simulink model "VFlexP"  (R2024a)
settings: Solver=ode23tb  StartTime=0.0  StopTime=3  FixedStep=1e-5
model workspace (MAT data in the model file):
  DCop_DCBUCK : object (value not decoded)
  Grid_CCVSC_idx = [2; 3; 4; 5; 6; 7; 8; 9; 10; 11; 12]
  Grid_CCVSCs = 1
  Grid_CCVSCs_buses = 1
  Grid_CCVSCs_toM = [0 1 0 0 0 0 0 0 0 0 0 0 ... (781 elements, 71x11)]
  Grid_C_Lines = [0 0]
  Grid_Cbuses = [0.00666666666667 0.00666666666667 0.00666666666667]
  Grid_DC : object (value not decoded)
  Grid_DCop_DCBUCK : object (value not decoded)
  Grid_DCop_DC_PES : object (value not decoded)
  Grid_DFIGs = 1
  Grid_DFIGs_buses = 1
  Grid_DGs : string (value not decoded)
  Grid_From_buses = [1 2]
  Grid_GFls = 1
  Grid_GFls_buses = 1
  Grid_GFr_idx = 1
  Grid_GFrs = 1
  Grid_GFrs_buses = 1
  Grid_GFrs_toM = [1; 0; 0]
  Grid_IG_idx = 2
  Grid_IGs = 1
  Grid_IGs_buses = 1
  Grid_IGs_toM = [0; 1]
  Grid_L_Lines = [0.05 0.05]
  Grid_L_Loads = 0
  Grid_Lines_fromM : object (value not decoded)
  Grid_Lines_toM : object (value not decoded)
  Grid_Load_buses = []
  Grid_Load_busesDC = []
  Grid_MSGs = 1
  Grid_MSGs_buses = 1
  Grid_Nbuses = 3
  Grid_PQ_gen = 3
  Grid_Ploads = []
  Grid_PloadsDC = []
  Grid_Ps_lf = -0.138475313333
  Grid_Qloads = []
  Grid_Qs_lf = 0.00594619333333
  Grid_R_Lines = [0.005 0.005]
  Grid_R_Loads = 0
  Grid_R_Loads_DC = 0
  Grid_Rcf = [150 150 150]
  Grid_SCs = 1
  Grid_SCs_buses = 1
  Grid_SG_idx = 1
  Grid_SGs = 1
  Grid_SGs_buses = 1
  Grid_SGs_toM = [1; 0]
  Grid_To_buses = [2 3]
  Grid_VCVSC_idx = [1; 2; 3; 4; 5; 6; 7; 8; 9; 10; 11; 12]
  Grid_VCVSCs = 1
  Grid_VCVSCs_buses = [1; 2; 3; 6; 8; 9; 12; 58; 59; 60; 63; 65]
  Grid_VCVSCs_toM = [1 0 0 0 0 0 0 0 0 0 0 0 ... (852 elements, 71x12)]
  Grid_VSM_idx = 2
  Grid_VSMs = 1
  Grid_VSMs_buses = 1
  Grid_VSMs_toM = [0; 1]
  Grid_admitt_matrix = [1.9801990198-19.801979198i  -1.9801980198+19.801980198i; -1.9801980198+19.801980198i  1.9801990198-19.801979198i]
  Grid_admitt_matrix_noloads = [1.9801990198-19.801979198i  -1.9801980198+19.801980198i; -1.9801980198+19.801980198i  1.9801990198-19.801979198i]
  Grid_bus = [1; 2; 3]
  Grid_busDC_complexity = 1
  Grid_busDC_complexity_PF = 2
  Grid_bus_complexity = [1 1 1]
  Grid_bus_complexity_PF = [1 1 1]
  Grid_buses_lf = 1
  Grid_conductance_matrix = 0.00666666666667
  Grid_conductance_matrix_noloads = 0.00666666666667
  Grid_fref : object (value not decoded)
  Grid_gen_static_params : mBase (value not decoded)
  Grid_iPs_lf = -7.22150378958
  Grid_iQs_lf = 168.17482109
  Grid_iadmitt_matrix = [250000.001075-249999.987531i  249999.998575-250000.012531i; 249999.998575-250000.012531i  250000.001075-249999.987531i]
  Grid_iadmitt_matrix_noloads = [250000.001075-249999.987531i  249999.998575-250000.012531i; 249999.998575-250000.012531i  250000.001075-249999.987531i]
  Grid_iconductance_matrix = 150
  Grid_iconductance_matrix_noloads = 150
  Grid_init_OK_bool = 1
  Grid_intconv_PF : object (value not decoded)
  Grid_lf_op : op_report (value not decoded)
  Grid_lineDC_complexity = []
  Grid_lineDC_complexity_PF = []
  Grid_line_complexity = [1 1]
  Grid_line_complexity_PF = [3 3]
  Grid_loadDC_complexity = []
  Grid_loadDC_complexity_PF = []
  Grid_load_complexity = []
  Grid_load_complexity_PF = []
  Grid_opDC_CCVSC : object (value not decoded)
  Grid_opDC_VSM : object (value not decoded)
  Grid_opGFr : object (value not decoded)
  Grid_opVCVSC : object (value not decoded)
  Grid_op_CCVSC : object (value not decoded)
  Grid_op_IG : object (value not decoded)
  Grid_op_SG : object (value not decoded)
  Grid_op_VSM : object (value not decoded)
  Grid_shift_lines = [0 0]
  Grid_tap_lines = [1 1]
  Grid_v_buses_mod = [1 1.0001218564 1]
  LinsysParamChangeStruct : Param1 (value not decoded)
  Lline = 0.01
  Rline = 1e-05
  linsys : object (value not decoded)
symbols that are objects in the model workspace (value not decoded): Grid_DCop_DC_PES, Grid_DCop_DCBUCK, Grid_op_CCVSC, Grid_op_IG, Grid_op_SG, Grid_op_VSM, Grid_opDC_CCVSC, Grid_opDC_VSM, Grid_opGFr, Grid_opVCVSC
undefined symbols (not defined in the file or in its folder): block_buses_DC, block_idx, CCVSC_idx, Cf, costs, costs2, DFIGs_nodes, DiscIntNeverNeededParam, entity, Fb, Fi, From_nodes, Grid_op_DFIG, Grid_op_DFIG_PQ, Grid_op_MSG, Grid_op_SC, Grid_op_VCVSC, Kic, Kiv, Kpc, Kpv, last_send, Lc, Lf, m, Matrix_flux_to_i, mD, mp, MSGs_buses, Nbuses_DC, nq, op_VCVSC, Psche, Rc, Rf, rkq1, rkq2, SCs_buses, SCs_nodes, sec_control_structure, set_DG_up, set_extra_satur, set_sending_cost, SGs_buses, SGs_nodes, Tf, To_nodes, VI_L, VI_R, WOF_Tf, xkq1, xkq2
libraries: simulink x447, eeGeneralControl x5
(part 19 of 30)

== system VFlexP/Grid/Dynamic/Grid/Dynamic/Loads/PQ ==
  v_in : Inport
  connected : Inport  Port=2
  iP : Inport  Port=3
  Constant : Constant  Value=Ploads(load_complexity == 4)/Sb  VectorParams1D=off
  Constant1 : Constant  Value=Qloads(load_complexity == 4)/Sb  VectorParams1D=off
  Constant2 : Constant  Value=Inf
  Constant3 : Constant  Value=zeros(1, sum(load_complexity == 4))  VectorParams1D=off
  Divide : Product  Inputs=*/
  Divide1 : Product  Inputs=*/
  For Each Subsystem : Subsystem  TreatAsAtomicUnit=on
  Gain : Gain  Gain=Ploads(load_complexity == 4)/Sb
  Matrix Concatenate : Concatenate  NumInputs=3  Mode=Multidimensional array
  Product{,1..7} (8 alike) : Product
  Selector : Selector  NumberOfDimensions=2  InputPortWidth=3  IndexOptions=Index vector (dialog),Index vector (dialog)  Indices=1,find(load_complexity == 4)  OutputSizes=1,1
  Selector1 : Selector  NumberOfDimensions=2  InputPortWidth=3  IndexOptions=Index vector (dialog),Index vector (dialog)  Indices=2,find(load_complexity == 4)  OutputSizes=1,1
  Selector2 : Selector  InputPortWidth=length(R_Loads)  IndexOptions=Index vector (dialog)  Indices=find(load_complexity == 4)  OutputSizes=1
  Selector3 : Selector  InputPortWidth=length(R_Loads)  IndexOptions=Index vector (dialog)  Indices=find(load_complexity == 4)  OutputSizes=1
  Sum : Sum  Inputs=|++
  Sum1 : Sum  Inputs=|+-
  Sum2 : Sum  Inputs=|++
  Sum4 : Sum  Inputs=|++
  Switch : Switch  Criteria=u2 > Threshold  Threshold=1e-5  ZeroCross=off  SaturateOnIntegerOverflow=off  InputSameDT=off
  i : Outport
  wires:
  Product1/1 -> Sum/2
  Product/1 -> Sum/1
  Sum2/1 -> Product/1, Product2/1  "Prefnew"
  Product2/1 -> Sum1/1
  v_in/1 -> Selector1/1, Selector/1
  Product3/1 -> Sum1/2
  Product5/1 -> Sum4/2
  Constant1/1 -> Product3/1, Product1/2  "Qrefnew"
  Product4/1 -> Sum4/1
  Sum/1 -> Divide/1
  Switch/1 -> Divide1/2, Divide/2
  Sum4/1 -> Switch/1, Switch/2
  Constant2/1 -> Switch/3
  Sum1/1 -> Divide1/1
  connected/1 -> Selector2/1
  Divide/1 -> Product6/2  "id"
  Divide1/1 -> Product7/2  "iqref"
  Selector/1 -> Product4/1, Product4/2, Product/2, Product3/2  "id1"
  Selector1/1 -> Product5/1, Product5/2, Product2/2, Product1/1  "iq1"
  Matrix Concatenate/1 -> For Each Subsystem/1(In1)
  Product6/1 -> Matrix Concatenate/1
  Product7/1 -> Matrix Concatenate/2
  Selector2/1 -> Product6/1, Product7/1
  For Each Subsystem/1(Out1) -> i/1
  Constant3/1 -> Matrix Concatenate/3
  Selector3/1 -> Gain/1
  Gain/1 -> Sum2/1
  iP/1 -> Selector3/1
  Constant/1 -> Sum2/2  "Prefnew"

== system VFlexP/Grid/Dynamic/Grid/Dynamic/Loads/dynamic PQ ==
  v_in : Inport
  connected : Inport  Port=2
  iP : Inport  Port=3
  Constant : Constant  Value=Ploads(load_complexity == 5)/Sb  VectorParams1D=off
  Constant1 : Constant  Value=Qloads(load_complexity == 5)/Sb  VectorParams1D=off
  Constant2 : Constant  Value=Inf
  Constant3 : Constant  Value=zeros(1, sum(load_complexity == 5))  VectorParams1D=off
  Divide : Product  Inputs=*/
  Divide1 : Product  Inputs=*/
  For Each Subsystem : Subsystem  TreatAsAtomicUnit=on
  Gain : Gain  Gain=Ploads(load_complexity == 5)/Sb
  Matrix Concatenate : Concatenate  NumInputs=3  Mode=Multidimensional array
  Product{,1..7} (8 alike) : Product
  Selector : Selector  NumberOfDimensions=2  InputPortWidth=3  IndexOptions=Index vector (dialog),Index vector (dialog)  Indices=1,find(load_complexity == 5)  OutputSizes=1,1
  Selector1 : Selector  NumberOfDimensions=2  InputPortWidth=3  IndexOptions=Index vector (dialog),Index vector (dialog)  Indices=2,find(load_complexity == 5)  OutputSizes=1,1
  Selector2 : Selector  InputPortWidth=length(R_Loads)  IndexOptions=Index vector (dialog)  Indices=find(load_complexity == 5)  OutputSizes=1
  Selector3 : Selector  InputPortWidth=length(R_Loads)  IndexOptions=Index vector (dialog)  Indices=find(load_complexity == 5)  OutputSizes=1
  Signal Specification : SignalSpecification  Dimensions=[3 sum(load_complexity == 5)]
  Sum : Sum  Inputs=|++
  Sum1 : Sum  Inputs=|+-
  Sum2 : Sum  Inputs=|++
  Sum4 : Sum  Inputs=|++
  Switch : Switch  Criteria=u2 > Threshold  Threshold=1e-5  ZeroCross=off  SaturateOnIntegerOverflow=off  InputSameDT=off
  i_d : Subsystem  mask{T_s=0.01}
      mask prompts: T_s "Filter time constant"
      mask Display:
      | try
      |     dpoly(1, [T_s, 1])
      | catch
      | end
  i_q : Subsystem  mask{T_s=0.01}
      mask prompts: T_s "Filter time constant"
      mask Display:
      | try
      |     dpoly(1, [T_s, 1])
      | catch
      | end
  i : Outport
  wires:
  Product7/1 -> i_q/1(in)
  Divide1/1 -> Product7/2  "iqref"
  Product6/1 -> i_d/1(in)
  Divide/1 -> Product6/2  "id"
  connected/1 -> Selector2/1
  Sum1/1 -> Divide1/1
  Constant2/1 -> Switch/3
  Sum4/1 -> Switch/2, Switch/1
  Switch/1 -> Divide/2, Divide1/2
  Sum/1 -> Divide/1
  Product4/1 -> Sum4/1
  Product5/1 -> Sum4/2
  Product3/1 -> Sum1/2
  v_in/1 -> Selector/1, Selector1/1
  Product2/1 -> Sum1/1
  Sum2/1 -> Product2/1, Product/1  "Prefnew"
  Product/1 -> Sum/1
  Product1/1 -> Sum/2
  iP/1 -> Selector3/1
  Constant/1 -> Sum2/2  "Prefnew"
  Gain/1 -> Sum2/1
  Constant1/1 -> Product1/2, Product3/1  "Qrefnew"
  Selector/1 -> Product3/2, Product/2, Product4/2, Product4/1  "id1"
  Selector1/1 -> Product1/1, Product2/2, Product5/2, Product5/1  "iq1"
  Matrix Concatenate/1 -> Signal Specification/1
  i_d/1(out) -> Matrix Concatenate/1
  i_q/1(out) -> Matrix Concatenate/2
  Selector2/1 -> Product7/1, Product6/1
  Selector3/1 -> Gain/1
  For Each Subsystem/1(Out1) -> i/1
  Signal Specification/1 -> For Each Subsystem/1(In1)
  Constant3/1 -> Matrix Concatenate/3

== system VFlexP/Grid/Dynamic/Grid/Dynamic/Loads/parallel RL dynamic ==
  v_in : Inport
  connected : Inport  Port=2
  Constant : Constant
  Constant1 : Constant  Value=zeros(1, sum(load_complexity == 6))  VectorParams1D=off
  For Each Subsystem : Subsystem  TreatAsAtomicUnit=on
  Gain1 : Gain  Gain=(v_buses_mod(Load_buses(load_complexity == 6)).^2)./Qloads(load_complexity == 6)*Sb
  Gain2 : Gain  Gain=(Ploads(load_complexity == 6)./v_buses_mod(Load_buses(load_complexity == 6)).^2)/Sb
  Gain3 : Gain  Gain=(Ploads(load_complexity == 6)./v_buses_mod(Load_buses(load_complexity == 6)).^2)/Sb
  Gain4 : Gain  Gain=(v_buses_mod(Load_buses(load_complexity == 6)).^2)./Qloads(load_complexity == 6)*Sb
  Gain5 : Gain  Gain=Qloads(load_complexity == 6)./(v_buses_mod(Load_buses(load_complexity == 6)).^2)/Sb
  Gain7 : Gain  Gain=Qloads(load_complexity == 6)./(v_buses_mod(Load_buses(load_complexity == 6)).^2)/Sb
  Matrix Concatenate : Concatenate  NumInputs=3  Mode=Multidimensional array
  Product{,1,6..9} (6 alike) : Product
  Selector : Selector  NumberOfDimensions=2  InputPortWidth=3  IndexOptions=Index vector (dialog),Index vector (dialog)  Indices=1,find(load_complexity == 6)  OutputSizes=1,1
  Selector1 : Selector  NumberOfDimensions=2  InputPortWidth=3  IndexOptions=Index vector (dialog),Index vector (dialog)  Indices=2,find(load_complexity == 6)  OutputSizes=1,1
  Selector3 : Selector  InputPortWidth=length(R_Loads)  IndexOptions=Index vector (dialog)  Indices=find(load_complexity == 6)  OutputSizes=1
  Selector4 : Selector  InputPortWidth=length(fref.ref_units)  IndexOptions=Index vector (dialog)  Indices=fref.loads(load_complexity == 6)  OutputSizes=1
  Selector8 : Selector  InputPortWidth=length(fref.ref_units)  IndexOptions=Index vector (dialog)  Indices=fref.loads(load_complexity == 6)  OutputSizes=1
  Signal Specification : SignalSpecification  Dimensions=[3 sum(load_complexity == 6)]
  Sum : Sum  Inputs=|++
  Sum1 : Sum  Inputs=|++
  Sum6 : Sum  Inputs=|++
  Sum8 : Sum  Inputs=|+-
  i_d : Integrator  InitialCondition=Grid_lf_op.op_report.Outputs(8).y(Load_buses(load_complexity == 6)).*Qloads(load_complexity == 6)./(v_buses_mod(Load_buses(load_complexity == 6)).^2)/Sb
  i_q : Integrator  InitialCondition=Grid_lf_op.op_report.Outputs(7).y(Load_buses(load_complexity == 6)).*-Qloads(load_complexity == 6)./(v_buses_mod(Load_buses(load_complexity == 6)).^2)/Sb
  i : Outport
  wires:
  Sum8/1 -> Gain7/1
  Selector4/1 -> Product/2, Product1/1
  [omega_ref] -> Selector4/1  "omega"
  Signal Specification/1 -> For Each Subsystem/1(In1)
  Selector/1 -> Product8/2
  Product6/1 -> i_d/1
  Selector1/1 -> Product9/2
  Selector3/1 -> Product8/1, Product9/1
  i_q/1 -> Sum1/1, Gain4/1  "iq"
  connected/1 -> Selector3/1
  [omega_base] -> Selector8/1
  For Each Subsystem/1(Out1) -> i/1
  Gain1/1 -> Product1/2
  Sum6/1 -> Gain5/1
  Product1/1 -> Sum8/2
  Gain7/1 -> Product7/2
  i_d/1 -> Sum/1, Gain1/1  "id"
  Gain4/1 -> Product/1
  v_in/1 -> Selector/1, Selector1/1
  Product7/1 -> i_q/1
  Constant1/1 -> Matrix Concatenate/3
  Product/1 -> Sum6/2
  Selector8/1 -> Product7/1, Product6/2
  Product9/1 -> Gain3/1, Sum8/1
  Product8/1 -> Gain2/1, Sum6/1
  Matrix Concatenate/1 -> Signal Specification/1
  Gain5/1 -> Product6/1
  Sum/1 -> Matrix Concatenate/1
  Gain2/1 -> Sum/2
  Gain3/1 -> Sum1/2
  Sum1/1 -> Matrix Concatenate/2

== system VFlexP/Grid/Dynamic/Grid/Dynamic/Loads/parallel RL static ==
  v_in : Inport
  connected : Inport  Port=2
  Constant : Constant  Value=R_Loads(load_complexity == 1)  VectorParams1D=off
  Constant1 : Constant  Value=zeros(1, sum(load_complexity == 1))  VectorParams1D=off
  For Each Subsystem : Subsystem  TreatAsAtomicUnit=on
  Gain1 : Gain  Gain=L_Loads(load_complexity == 1)
  Gain4 : Gain  Gain=L_Loads(load_complexity == 1)
  Gain5 : Gain  Gain=1./L_Loads(load_complexity == 1)
  Gain7 : Gain  Gain=1./L_Loads(load_complexity == 1)
  Matrix Concatenate : Concatenate  NumInputs=3  Mode=Multidimensional array
  Product{,1,4..9} (8 alike) : Product
  Selector : Selector  NumberOfDimensions=2  InputPortWidth=3  IndexOptions=Index vector (dialog),Index vector (dialog)  Indices=1,find(load_complexity == 1)  OutputSizes=1,1
  Selector1 : Selector  NumberOfDimensions=2  InputPortWidth=3  IndexOptions=Index vector (dialog),Index vector (dialog)  Indices=2,find(load_complexity == 1)  OutputSizes=1,1
  Selector3 : Selector  InputPortWidth=length(R_Loads)  IndexOptions=Index vector (dialog)  Indices=find(load_complexity == 1)  OutputSizes=1
  Selector4 : Selector  InputPortWidth=length(fref.ref_units)  IndexOptions=Index vector (dialog)  Indices=fref.loads(load_complexity == 1)  OutputSizes=1
  Selector8 : Selector  InputPortWidth=length(fref.ref_units)  IndexOptions=Index vector (dialog)  Indices=fref.loads(load_complexity == 1)  OutputSizes=1
  Signal Specification : SignalSpecification  Dimensions=[3 sum(load_complexity == 1)]
  Sum4 : Sum  Inputs=+-|
  Sum5 : Sum  Inputs=|-+
  Sum6 : Sum  Inputs=|++
  Sum7 : Sum  Inputs=-+|
  Sum8 : Sum  Inputs=|+-
  Sum9 : Sum  Inputs=-+|
  Zero : Constant  Value=0  OutDataTypeStr=Inherit: Inherit via back propagation
  Zero1 : Constant  Value=0  OutDataTypeStr=Inherit: Inherit via back propagation
  i_d : Integrator  InitialCondition=Grid_lf_op.op_report.Outputs(5).y(load_complexity == 1)
  i_q : Integrator  InitialCondition=Grid_lf_op.op_report.Outputs(6).y(load_complexity == 1)
  i : Outport
  wires:
  v_in/1 -> Selector1/1, Selector/1
  Product5/1 -> Sum4/2
  i_d/1 -> Matrix Concatenate/1, Gain1/1, Product5/1  "id"
  Sum6/1 -> Gain5/1
  [omega_ref] -> Selector4/1  "omega"
  Product/1 -> Sum6/2
  Sum8/1 -> Gain7/1
  Sum4/1 -> Sum7/2
  Product1/1 -> Sum8/2
  Gain4/1 -> Product/1
  Sum7/1 -> Sum6/1
  Product4/1 -> Sum5/1
  Sum5/1 -> Sum9/2
  i_q/1 -> Matrix Concatenate/2, Product4/1, Gain4/1  "iq"
  Gain1/1 -> Product1/2
  Sum9/1 -> Sum8/1
  Zero/1 -> Sum7/1  "v_out_d"
  Zero1/1 -> Sum9/1  "v_out_q"
  Matrix Concatenate/1 -> Signal Specification/1
  Product8/1 -> Sum4/1  "id1"
  Product9/1 -> Sum5/2  "iq1"
  For Each Subsystem/1(Out1) -> i/1
  Signal Specification/1 -> For Each Subsystem/1(In1)
  Constant1/1 -> Matrix Concatenate/3
  Constant/1 -> Product5/2, Product4/2  "R"
  Selector4/1 -> Product1/1, Product/2
  [omega_base] -> Selector8/1
  Selector8/1 -> Product6/2, Product7/1
  Product7/1 -> i_q/1
  Gain7/1 -> Product7/2
  Gain5/1 -> Product6/1
  Product6/1 -> i_d/1
  connected/1 -> Selector3/1
  Selector/1 -> Product8/2  "id1"
  Selector3/1 -> Product9/1, Product8/1
  Selector1/1 -> Product9/2  "iq1"

== system VFlexP/Grid/Dynamic/Grid/Dynamic/Loads/parallel RL static omega ==
  v_in : Inport
  connected : Inport  Port=2
  Constant : Constant  Value=R_Loads(load_complexity == 1)  VectorParams1D=off
  Constant1 : Constant  Value=zeros(1, sum(load_complexity == 1))  VectorParams1D=off
  For Each Subsystem : Subsystem  TreatAsAtomicUnit=on
  Gain1 : Gain  Gain=L_Loads(load_complexity == 1)
  Gain4 : Gain  Gain=L_Loads(load_complexity == 1)
  Gain5 : Gain  Gain=1./L_Loads(load_complexity == 1)
  Gain7 : Gain  Gain=1./L_Loads(load_complexity == 1)
  Matrix Concatenate : Concatenate  NumInputs=3  Mode=Multidimensional array
  Product{,1,4..9} (8 alike) : Product
  Selector : Selector  NumberOfDimensions=2  InputPortWidth=3  IndexOptions=Index vector (dialog),Index vector (dialog)  Indices=1,find(load_complexity == 1)  OutputSizes=1,1
  Selector1 : Selector  NumberOfDimensions=2  InputPortWidth=3  IndexOptions=Index vector (dialog),Index vector (dialog)  Indices=2,find(load_complexity == 1)  OutputSizes=1,1
  Selector3 : Selector  InputPortWidth=length(R_Loads)  IndexOptions=Index vector (dialog)  Indices=find(load_complexity == 1)  OutputSizes=1
  Selector4 : Selector  InputPortWidth=length(fref.ref_units)  IndexOptions=Index vector (dialog)  Indices=fref.loads(load_complexity == 1)  OutputSizes=1
  Selector8 : Selector  InputPortWidth=length(fref.ref_units)  IndexOptions=Index vector (dialog)  Indices=fref.loads(load_complexity == 1)  OutputSizes=1
  Signal Specification : SignalSpecification  Dimensions=[3 sum(load_complexity == 1)]
  Sum4 : Sum  Inputs=+-|
  Sum5 : Sum  Inputs=|-+
  Sum6 : Sum  Inputs=|++
  Sum7 : Sum  Inputs=-+|
  Sum8 : Sum  Inputs=|+-
  Sum9 : Sum  Inputs=-+|
  Zero : Constant  Value=0  OutDataTypeStr=Inherit: Inherit via back propagation
  Zero1 : Constant  Value=0  OutDataTypeStr=Inherit: Inherit via back propagation
  i_d : Integrator  InitialCondition=Grid_lf_op.op_report.Outputs(5).y(load_complexity == 1)
  i_q : Integrator  InitialCondition=Grid_lf_op.op_report.Outputs(6).y(load_complexity == 1)
  i : Outport
  wires:
  Selector1/1 -> Product9/2  "iq1"
  Selector3/1 -> Product8/1, Product9/1
  Selector/1 -> Product8/2  "id1"
  connected/1 -> Selector3/1
  Product6/1 -> i_d/1
  Gain5/1 -> Product6/1
  Gain7/1 -> Product7/2
  Product7/1 -> i_q/1
  Selector8/1 -> Product7/1, Product6/2
  [omega_base] -> Selector8/1
  Selector4/1 -> Product/2, Product1/1
  Constant/1 -> Product4/2, Product5/2  "R"
  Constant1/1 -> Matrix Concatenate/3
  Signal Specification/1 -> For Each Subsystem/1(In1)
  For Each Subsystem/1(Out1) -> i/1
  Product9/1 -> Sum5/2  "iq1"
  Product8/1 -> Sum4/1  "id1"
  Matrix Concatenate/1 -> Signal Specification/1
  Zero1/1 -> Sum9/1  "v_out_q"
  Zero/1 -> Sum7/1  "v_out_d"
  Sum9/1 -> Sum8/1
  Gain1/1 -> Product1/2
  i_q/1 -> Gain4/1, Product4/1, Matrix Concatenate/2  "iq"
  Sum5/1 -> Sum9/2
  Product4/1 -> Sum5/1
  Sum7/1 -> Sum6/1
  Gain4/1 -> Product/1
  Product1/1 -> Sum8/2
  Sum4/1 -> Sum7/2
  Sum8/1 -> Gain7/1
  Product/1 -> Sum6/2
  [omega_ref] -> Selector4/1  "omega"
  Sum6/1 -> Gain5/1
  i_d/1 -> Product5/1, Gain1/1, Matrix Concatenate/1  "id"
  Product5/1 -> Sum4/2
  v_in/1 -> Selector/1, Selector1/1

== system VFlexP/Grid/Dynamic/Grid/Dynamic/Loads/series RL dynamic ==
  v_in : Inport
  connected : Inport  Port=2
  Constant : Constant  Value=R_Loads(load_complexity == 1)  VectorParams1D=off
  Constant1 : Constant  Value=zeros(1, sum(load_complexity == 1))  VectorParams1D=off
  For Each Subsystem : Subsystem  TreatAsAtomicUnit=on
  Gain1 : Gain  Gain=L_Loads(load_complexity == 1)
  Gain4 : Gain  Gain=L_Loads(load_complexity == 1)
  Gain5 : Gain  Gain=1./L_Loads(load_complexity == 1)
  Gain7 : Gain  Gain=1./L_Loads(load_complexity == 1)
  Matrix Concatenate : Concatenate  NumInputs=3  Mode=Multidimensional array
  Product{,1,4..9} (8 alike) : Product
  Selector : Selector  NumberOfDimensions=2  InputPortWidth=3  IndexOptions=Index vector (dialog),Index vector (dialog)  Indices=1,find(load_complexity == 1)  OutputSizes=1,1
  Selector1 : Selector  NumberOfDimensions=2  InputPortWidth=3  IndexOptions=Index vector (dialog),Index vector (dialog)  Indices=2,find(load_complexity == 1)  OutputSizes=1,1
  Selector3 : Selector  InputPortWidth=length(R_Loads)  IndexOptions=Index vector (dialog)  Indices=find(load_complexity == 1)  OutputSizes=1
  Selector4 : Selector  InputPortWidth=length(fref.ref_units)  IndexOptions=Index vector (dialog)  Indices=fref.loads(load_complexity == 1)  OutputSizes=1
  Selector8 : Selector  InputPortWidth=length(fref.ref_units)  IndexOptions=Index vector (dialog)  Indices=fref.loads(load_complexity == 1)  OutputSizes=1
  Signal Specification : SignalSpecification  Dimensions=[3 sum(load_complexity == 1)]
  Sum4 : Sum  Inputs=+-|
  Sum5 : Sum  Inputs=|-+
  Sum6 : Sum  Inputs=|++
  Sum7 : Sum  Inputs=-+|
  Sum8 : Sum  Inputs=|+-
  Sum9 : Sum  Inputs=-+|
  Zero : Constant  Value=0  OutDataTypeStr=Inherit: Inherit via back propagation
  Zero1 : Constant  Value=0  OutDataTypeStr=Inherit: Inherit via back propagation
  i_d : Integrator  InitialCondition=Grid_lf_op.op_report.Outputs(5).y(load_complexity == 1)
  i_q : Integrator  InitialCondition=Grid_lf_op.op_report.Outputs(6).y(load_complexity == 1)
  i : Outport
  wires:
  v_in/1 -> Selector1/1, Selector/1
  Product5/1 -> Sum4/2
  i_d/1 -> Matrix Concatenate/1, Gain1/1, Product5/1  "id"
  Sum6/1 -> Gain5/1
  [omega_ref] -> Selector4/1  "omega"
  Product/1 -> Sum6/2
  Sum8/1 -> Gain7/1
  Sum4/1 -> Sum7/2
  Product1/1 -> Sum8/2
  Gain4/1 -> Product/1
  Sum7/1 -> Sum6/1
  Product4/1 -> Sum5/1
  Sum5/1 -> Sum9/2
  i_q/1 -> Matrix Concatenate/2, Product4/1, Gain4/1  "iq"
  Gain1/1 -> Product1/2
  Sum9/1 -> Sum8/1
  Zero/1 -> Sum7/1  "v_out_d"
  Zero1/1 -> Sum9/1  "v_out_q"
  Matrix Concatenate/1 -> Signal Specification/1
  Product8/1 -> Sum4/1  "id1"
  Product9/1 -> Sum5/2  "iq1"
  For Each Subsystem/1(Out1) -> i/1
  Signal Specification/1 -> For Each Subsystem/1(In1)
  Constant1/1 -> Matrix Concatenate/3
  Constant/1 -> Product5/2, Product4/2  "R"
  Selector4/1 -> Product1/1, Product/2
  [omega_base] -> Selector8/1
  Selector8/1 -> Product6/2, Product7/1
  Gain7/1 -> Product7/2
  Gain5/1 -> Product6/1
  connected/1 -> Selector3/1
  Selector/1 -> Product8/2  "id1"
  Selector3/1 -> Product9/1, Product8/1
  Selector1/1 -> Product9/2  "iq1"
  Product6/1 -> i_d/1
  Product7/1 -> i_q/1

== system VFlexP/Grid/Dynamic/Grid/Dynamic/Loads/series RL static ==
  connected : Inport
  v_in : Inport  Port=2
  Constant : Constant  Value=R_Loads(load_complexity == 2)  VectorParams1D=off
  Constant1 : Constant
  Constant2 : Constant  Value=zeros(1, sum(load_complexity == 2))  VectorParams1D=off
  Divide : Product  Inputs=*/
  For Each Subsystem : Subsystem  TreatAsAtomicUnit=on
  Gain : Gain  Gain=L_Loads(load_complexity == 2)
  Gain1 : Gain  Gain=R_Loads(load_complexity == 2)
  Gain2 : Gain  Gain=R_Loads(load_complexity == 2)
  Matrix Concatenate : Concatenate  NumInputs=3  Mode=Multidimensional array
  Product{,1..7} (8 alike) : Product
  Selector : Selector  NumberOfDimensions=2  InputPortWidth=3  IndexOptions=Index vector (dialog),Index vector (dialog)  Indices=1,find(load_complexity == 2)  OutputSizes=1,1
  Selector1 : Selector  NumberOfDimensions=2  InputPortWidth=3  IndexOptions=Index vector (dialog),Index vector (dialog)  Indices=2,find(load_complexity == 2)  OutputSizes=1,1
  Selector2 : Selector  InputPortWidth=length(R_Loads)  IndexOptions=Index vector (dialog)  Indices=find(load_complexity == 2)  OutputSizes=1
  Selector4 : Selector  InputPortWidth=length(fref.ref_units)  IndexOptions=Index vector (dialog)  Indices=fref.loads(load_complexity == 2)  OutputSizes=1
  Sum : Sum  Inputs=|++
  Sum1 : Sum  Inputs=|+-
  Sum2 : Sum  Inputs=|+-
  Sum3 : Sum  Inputs=|++
  Sum4 : Sum  Inputs=|-+
  Zero : Constant  Value=0  OutDataTypeStr=Inherit: Inherit via back propagation
  Zero1 : Constant  Value=0  OutDataTypeStr=Inherit: Inherit via back propagation
  i : Outport
  wires:
  v_in/1 -> Selector1/1, Selector/1
  Zero/1 -> Sum1/2  "v_out_d"
  Sum/1 -> Divide/2
  Gain2/1 -> Product5/2
  Product/1 -> Sum/2
  Product1/1 -> Sum3/1
  Product5/1 -> Sum4/2
  Sum2/1 -> Product3/2, Product5/1  "vq"
  Gain/1 -> Product2/2, Product/1, Product/2
  Constant1/1 -> Divide/1
  Product3/1 -> Sum3/2
  Sum1/1 -> Product4/1, Product1/1  "vd"
  Divide/1 -> Product2/1, Gain1/1, Gain2/1
  Product4/1 -> Sum4/1
  Product2/1 -> Product3/1, Product4/2
  Gain1/1 -> Product1/2
  Zero1/1 -> Sum2/2  "v_out_q"
  [omega_ref] -> Selector4/1  "omega"
  connected/1 -> Selector2/1
  Sum3/1 -> Product6/2  "id"
  Sum4/1 -> Product7/2
  Product7/1 -> Matrix Concatenate/2
  Selector/1 -> Sum1/1  "id1"
  Selector1/1 -> Sum2/1  "iq1"
  Matrix Concatenate/1 -> For Each Subsystem/1(In1)
  Product6/1 -> Matrix Concatenate/1
  Selector2/1 -> Product6/1, Product7/1
  For Each Subsystem/1(Out1) -> i/1
  Constant2/1 -> Matrix Concatenate/3
  Constant/1 -> Sum/1
  Selector4/1 -> Gain/1

== system VFlexP/Grid/Dynamic/Grid/Dynamic/Loads/series RL static omega ==
  v_in : Inport
  connected : Inport  Port=2
  Constant1 : Constant  Value=zeros(1, sum(load_complexity == 3))  VectorParams1D=off
  For Each Subsystem : Subsystem  TreatAsAtomicUnit=on
  Gain : Gain  Gain=1./(R_Loads(load_complexity == 3).^2+L_Loads(load_complexity == 3).^2)
  Gain2 : Gain  Gain=1./(R_Loads(load_complexity == 3).^2+L_Loads(load_complexity == 3).^2)
  Gain3 : Gain  Gain=R_Loads(load_complexity == 3)
  Gain4 : Gain  Gain=L_Loads(load_complexity == 3)
  Gain5 : Gain  Gain=L_Loads(load_complexity == 3)
  Gain6 : Gain  Gain=R_Loads(load_complexity == 3)
  Matrix Concatenate : Concatenate  NumInputs=3  Mode=Multidimensional array
  Product2 : Product
  Product3 : Product
  Selector : Selector  NumberOfDimensions=2  InputPortWidth=3  IndexOptions=Index vector (dialog),Index vector (dialog)  Indices=1,find(load_complexity == 3)  OutputSizes=1,1
  Selector1 : Selector  NumberOfDimensions=2  InputPortWidth=3  IndexOptions=Index vector (dialog),Index vector (dialog)  Indices=2,find(load_complexity == 3)  OutputSizes=1,1
  Selector2 : Selector  InputPortWidth=length(R_Loads)  IndexOptions=Index vector (dialog)  Indices=find(load_complexity == 3)  OutputSizes=1
  Sum : Sum  Inputs=|++
  Sum3 : Sum  Inputs=|-+
  i : Outport
  wires:
  Gain6/1 -> Sum3/2
  Gain5/1 -> Sum3/1
  Gain2/1 -> Gain4/1, Gain6/1
  Gain4/1 -> Sum/2
  Gain3/1 -> Sum/1
  Gain/1 -> Gain3/1, Gain5/1
  v_in/1 -> Selector1/1, Selector/1
  connected/1 -> Selector2/1
  Sum/1 -> Product2/2  "id"
  Sum3/1 -> Product3/2
  Selector/1 -> Gain/1  "id1"
  Selector1/1 -> Gain2/1  "iq1"
  Matrix Concatenate/1 -> For Each Subsystem/1(In1)
  Product3/1 -> Matrix Concatenate/2
  Product2/1 -> Matrix Concatenate/1
  Selector2/1 -> Product2/1, Product3/1
  For Each Subsystem/1(Out1) -> i/1
  Constant1/1 -> Matrix Concatenate/3

== system VFlexP/Grid/Dynamic/Grid/Dynamic/Loads to buses/LoadsM ==
  i : Inport  Partition=on  PartitionDimension=1  PartitionWidth=1  PartitionOffset=0
  Assignment : Assignment  DiagnosticForDimensions=Warning  IndexOptions=Index vector (dialog)  Indices=Load_buses  OutputSizes=1
  For Each : ForEach  DisableCoverage=on
  Zero : Constant  Value=zeros(1,Nbuses)  VectorParams1D=off  OutDataTypeStr=Inherit: Inherit via back propagation
  Out1 : Outport  ConcatenationDimension=1
  wires:
  Assignment/1 -> Out1/1
  i/1 -> Assignment/2
  Zero/1 -> Assignment/1

== system VFlexP/Grid/Dynamic/Grid/Dynamic/iCbuses/Subsystem ==
  In1 : Inport
  State-Space : StateSpace  A=[]  B=[]  C=[]  D=Lines_toM  InitialCondition=0  ParameterTunability=Optimized
  State-Space1 : StateSpace  A=[]  B=[]  C=[]  D=Lines_fromM  InitialCondition=0  ParameterTunability=Optimized
  Sum : Sum  Inputs=|++
  Transpose : Math  Operator=transpose
  Transpose1 : Math  Operator=transpose
  Transpose2 : Math  Operator=transpose
  Out1 : Outport
  wires:
  Transpose1/1 -> Sum/1
  State-Space1/1 -> Transpose2/1
  State-Space/1 -> Transpose1/1
  Transpose/1 -> State-Space1/1, State-Space/1
  Sum/1 -> Out1/1
  Transpose2/1 -> Sum/2
  In1/1 -> Transpose/1

== system VFlexP/Grid/Dynamic/Grid_DC/dynamic/BusesDC/dynamic ==
  i_in : Inport
  i_out : Inport  Port=2
  Gain1 : Gain  Gain=1/1e-1
  Gain2 : Gain  Gain=1./DC.Rbus(busDC_complexity == 1)';
  I1 : Integrator  InitialCondition=DC.v(busDC_complexity == 1)
  Scope : Scope
  Sum4 : Sum  Inputs=-+|
  Sum6 : Sum  Inputs=|+-
  v : Outport
  wires:
  Gain2/1 -> Sum4/1
  I1/1 -> Scope/1, v/1, Gain2/1
  i_in/1 -> Sum6/1
  Sum4/1 -> Gain1/1
  Sum6/1 -> Sum4/2
  i_out/1 -> Sum6/2
  Gain1/1 -> I1/1

== system VFlexP/Grid/Dynamic/Grid_DC/dynamic/BusesDC/static ==
  i_in : Inport
  i_out : Inport  Port=2
  Gain : Gain  Gain=1/1e-6
  LPF_d1 : Subsystem
  Sum1 : Sum  Inputs=+-
  v : Outport
  wires:
  Sum1/1 -> Gain/1
  i_in/1 -> Sum1/1
  i_out/1 -> Sum1/2
  Gain/1 -> LPF_d1/1(In1)
  LPF_d1/1(v_buses_dc) -> v/1

== system VFlexP/Grid/Dynamic/Grid_DC/dynamic/DClines/Dynamic ==
  V_dc_In : Inport
  V_dc_Out : Inport  Port=2
  1/L_dc : Gain  Gain=1./DC.L_Lines(lineDC_complexity == 1)
  For Each Subsystem : Subsystem  TreatAsAtomicUnit=on
  Integrator : Integrator  InitialCondition=DC.i_branch(lineDC_complexity_PF == 1)
  R_dc : Gain  Gain=DC.R_Lines(lineDC_complexity == 1)
  Selector : Selector  NumberOfDimensions=2  InputPortWidth=3  IndexOptions=Index vector (dialog),Index vector (dialog)  Indices=1,find(lineDC_complexity == 1)  OutputSizes=1,1
  Selector1 : Selector  NumberOfDimensions=2  InputPortWidth=3  IndexOptions=Index vector (dialog),Index vector (dialog)  Indices=1,find(lineDC_complexity == 1)  OutputSizes=1,1
  Sum4 : Sum  Inputs=-+-
  i : Outport
  wires:
  Integrator/1 -> For Each Subsystem/1(In1), R_dc/1
  Sum4/1 -> 1/L_dc/1
  1/L_dc/1 -> Integrator/1
  R_dc/1 -> Sum4/1
  For Each Subsystem/1(i) -> i/1
  V_dc_Out/1 -> Selector1/1
  V_dc_In/1 -> Selector/1
  Selector/1 -> Sum4/2
  Selector1/1 -> Sum4/3

== system VFlexP/Grid/Dynamic/Grid_DC/dynamic/DClines/Static ==
  V_dc_In : Inport
  V_dc_Out : Inport  Port=2
  For Each Subsystem : Subsystem  TreatAsAtomicUnit=on
  R_dc1 : Gain  Gain=1./DC.R_Lines(lineDC_complexity == 2)
  Selector : Selector  NumberOfDimensions=2  InputPortWidth=3  IndexOptions=Index vector (dialog),Index vector (dialog)  Indices=1,find(lineDC_complexity == 2)  OutputSizes=1,1
  Selector1 : Selector  NumberOfDimensions=2  InputPortWidth=3  IndexOptions=Index vector (dialog),Index vector (dialog)  Indices=1,find(lineDC_complexity == 2)  OutputSizes=1,1
  Sum4 : Sum  Inputs=+-
  i : Outport
  wires:
  Sum4/1 -> R_dc1/1
  R_dc1/1 -> For Each Subsystem/1(In1)
  For Each Subsystem/1(i) -> i/1
  V_dc_In/1 -> Selector/1
  Selector/1 -> Sum4/1
  V_dc_Out/1 -> Selector1/1
  Selector1/1 -> Sum4/2

== system VFlexP/Grid/Dynamic/Grid_DC/dynamic/Loads/ConstI ==
  connected : Inport
  Constant : Constant  Value=PloadsDC(loadDC_complexity == 3)/(Sb)
  Constant1 : Constant  Value=DC.v(loadDC_complexity == 3)
  Divide : Product  Inputs=*/
  For Each Subsystem : Subsystem  TreatAsAtomicUnit=on
  Product : Product
  Selector2 : Selector  InputPortWidth=length(R_Loads_DC)  IndexOptions=Index vector (dialog)  Indices=find(loadDC_complexity == 3)  OutputSizes=1
  i : Outport
  wires:
  connected/1 -> Selector2/1
  Selector2/1 -> Product/2
  Product/1 -> For Each Subsystem/1(In1)
  For Each Subsystem/1(i) -> i/1
  Constant/1 -> Divide/1
  Constant1/1 -> Divide/2
  Divide/1 -> Product/1

== system VFlexP/Grid/Dynamic/Grid_DC/dynamic/Loads/ConstP ==
  v_in : Inport
  connected : Inport  Port=2
  Constant : Constant  Value=PloadsDC(loadDC_complexity == 2)/Sb  VectorParams1D=off
  Divide : Product  Inputs=*/
  For Each Subsystem : Subsystem  TreatAsAtomicUnit=on
  Product : Product
  Selector : Selector  NumberOfDimensions=2  InputPortWidth=3  IndexOptions=Index vector (dialog),Index vector (dialog)  Indices=1,find(loadDC_complexity == 2)  OutputSizes=1,1
  Selector2 : Selector  InputPortWidth=length(R_Loads_DC)  IndexOptions=Index vector (dialog)  Indices=find(loadDC_complexity == 2)  OutputSizes=1
  i : Outport
  wires:
  Constant/1 -> Divide/1
  Divide/1 -> Product/1
  connected/1 -> Selector2/1
  Selector2/1 -> Product/2
  v_in/1 -> Selector/1
  Selector/1 -> Divide/2
  Product/1 -> For Each Subsystem/1(In1)
  For Each Subsystem/1(i) -> i/1

== system VFlexP/Grid/Dynamic/Grid_DC/dynamic/Loads/ConstR ==
  v_in : Inport
  connected : Inport  Port=2
  For Each Subsystem : Subsystem  TreatAsAtomicUnit=on
  Gain3 : Gain  Gain=1./R_Loads_DC(loadDC_complexity == 1)
  Product : Product
  Selector : Selector  NumberOfDimensions=2  InputPortWidth=3  IndexOptions=Index vector (dialog),Index vector (dialog)  Indices=1,find(loadDC_complexity == 1)  OutputSizes=1,1
  Selector2 : Selector  InputPortWidth=length(R_Loads_DC)  IndexOptions=Index vector (dialog)  Indices=find(loadDC_complexity == 1)  OutputSizes=1
  i : Outport
  wires:
  Gain3/1 -> Product/1
  connected/1 -> Selector2/1
  Selector2/1 -> Product/2
  v_in/1 -> Selector/1
  Selector/1 -> Gain3/1
  Product/1 -> For Each Subsystem/1(In1)
  For Each Subsystem/1(i) -> i/1

== system VFlexP/Grid/Dynamic/Grid_DC/dynamic/Loads/DynamicP ==
  v_in : Inport
  connected : Inport  Port=2
  Constant : Constant  Value=PloadsDC(loadDC_complexity == 4)/Sb
  For Each Subsystem : Subsystem  TreatAsAtomicUnit=on
  PI_Load : Subsystem
  Product : Product
  Product1 : Product
  Product2 : Product
  Selector : Selector  NumberOfDimensions=2  InputPortWidth=3  IndexOptions=Index vector (dialog),Index vector (dialog)  Indices=1,find(loadDC_complexity == 4)  OutputSizes=1,1
  Selector2 : Selector  InputPortWidth=length(R_Loads_DC)  IndexOptions=Index vector (dialog)  Indices=find(loadDC_complexity == 4)  OutputSizes=1
  Sum : Sum  Inputs=|+-
  i : Outport
  wires:
  Selector/1 -> Product2/1, Product1/1
  v_in/1 -> Selector/1
  Selector2/1 -> Product/2
  Constant/1 -> Sum/1
  connected/1 -> Selector2/1
  Product2/1 -> Sum/2
  Product1/1 -> Product/1, Product2/2
  For Each Subsystem/1(i) -> i/1
  Product/1 -> For Each Subsystem/1(In1)
  PI_Load/1(G_out) -> Product1/2
  Sum/1 -> PI_Load/1(e)

== system VFlexP/Grid/Dynamic/Grid_DC/dynamic/Loads to buses/LoadsM ==
  i : Inport  Partition=on  PartitionDimension=1  PartitionWidth=1  PartitionOffset=0
  Assignment : Assignment  DiagnosticForDimensions=Warning  IndexOptions=Index vector (dialog)  Indices=Load_busesDC  OutputSizes=1
  For Each : ForEach  DisableCoverage=on
  Zero : Constant  Value=zeros(1,DC.Nbuses)  VectorParams1D=off  OutDataTypeStr=Inherit: Inherit via back propagation
  i_out_buses : Outport  ConcatenationDimension=1
  wires:
  Assignment/1 -> i_out_buses/1
  i/1 -> Assignment/2
  Zero/1 -> Assignment/1

== system VFlexP/Grid/Dynamic/Secondary Control/MAS messages/ID1/Compare to last ==
  Output : Inport
  In4 : Inport  Port=2
  In1 : Inport  Port=3
  Output1 : Inport  Port=4
  time_last : Inport  Port=5
  com : Inport  Port=6
  AND : Logic  Inputs=3  IconShape=distinctive  AllPortsSameDT=off  OutDataTypeStr=boolean
  Abs : Abs  ZeroCross=off  SaturateOnIntegerOverflow=off
  Abs1 : Abs  ZeroCross=off  SaturateOnIntegerOverflow=off
  Clock1 : Clock
  Compare To Constant1 : simulink/Logic and Bit Operations/Compare To Constant  relop=>  const=1  OutDataTypeStr=boolean  ZeroCross=off
  Compare To Constant2 : simulink/Logic and Bit Operations/Compare To Constant  relop=>  const=1e-2  OutDataTypeStr=boolean  ZeroCross=off
  Gain : Gain  Gain=1e2
  Gain1 : Gain  Gain=1e2
  Send1 : Send  OutputPortMessageModes=m  ShowEnablePort=on
      settings: InputPortMap=e0,u1
  Sum : Sum  Inputs=|+-
  Sum1 : Sum  Inputs=|+-
  Sum2 : Sum  Inputs=|++
  Sum5 : Sum  Inputs=|+-
  Trigger : Outport
  wires:
  com/1 -> AND/3
  Gain1/1 -> Sum2/2
  Gain/1 -> Sum2/1
  Compare To Constant1/1 -> AND/1
  Sum2/1 -> Compare To Constant1/1
  Abs1/1 -> Gain1/1
  Compare To Constant2/1 -> AND/2
  Clock1/1 -> Sum1/1  "time"
  time_last/1 -> Sum1/2  "time_last"
  Sum1/1 -> Compare To Constant2/1
  AND/1 -> Send1/2, Send1/1
  In4/1 -> Sum5/2  "last_omega"
  Sum5/1 -> Abs1/1
  Abs/1 -> Gain/1
  Sum/1 -> Abs/1
  Send1/1 -> Trigger/1
  Output1/1 -> Sum5/1  "omega"
  In1/1 -> Sum/1  "v"
  Output/1 -> Sum/2  "last_v"

== system VFlexP/Grid/Dynamic/Secondary Control/MAS messages/ID1/Send to neighbor ==
  note: 1) Add Subsystem or Model blocks as valid variant choices.
      | 2) You cannot connect blocks at this level. At simulation, connectivity is automatically
      | determined, based on the active variant and port name matching.
  Message : Inport
  five : Subsystem  VariantControl=five
  four : Subsystem  VariantControl=four
  one : Subsystem  VariantControl=one
  three : Subsystem  VariantControl=three
  two : Subsystem  VariantControl=two

== system VFlexP/Grid/Dynamic/Secondary Control/MAS messages/ID1/Send to neighbor1 ==
  note: 1) Add Subsystem or Model blocks as valid variant choices.
      | 2) You cannot connect blocks at this level. At simulation, connectivity is automatically
      | determined, based on the active variant and port name matching.
  Message : Inport
  five : Subsystem  VariantControl=five
  four : Subsystem  VariantControl=four
  one : Subsystem  VariantControl=one
  three : Subsystem  VariantControl=three
  two : Subsystem  VariantControl=two

== system VFlexP/Grid/Dynamic/Secondary Control/MAS messages/ID1/Send to neighbor2 ==
  note: 1) Add Subsystem or Model blocks as valid variant choices.
      | 2) You cannot connect blocks at this level. At simulation, connectivity is automatically
      | determined, based on the active variant and port name matching.
  Message : Inport
  five : Subsystem  VariantControl=five
  four : Subsystem  VariantControl=four
  one : Subsystem  VariantControl=one
  three : Subsystem  VariantControl=three
  two : Subsystem  VariantControl=two

== system VFlexP/Grid/Dynamic/Secondary Control/MAS messages/ID1/Simulink Function ==
  Input : Inport
  get_cost : TriggerPort  TriggerType=function-call  IsSimulinkFunction=on  FunctionName=get_cost  FunctionVisibility=scoped  VariantControl=(inherit)
  y : ArgOut  DisableCoverage=on  ArgumentName=y
  wires:
  Input/1 -> y/1

== system VFlexP/Grid/Dynamic/Secondary Control/MAS messages/ID1/Simulink Function1 ==
  Input1 : Inport
  Input2 : Inport  Port=2
  Input3 : Inport  Port=3
  Input4 : Inport  Port=4
  Input6 : Inport  Port=5
  Input5 : Inport  Port=6
  Input7 : Inport  Port=7
  Output : Inport  Port=8
  In9 : Inport  Port=9
  In10 : Inport  Port=10
  package : TriggerPort  TriggerType=function-call  IsSimulinkFunction=on  FunctionName=package  FunctionVisibility=scoped  VariantControl=(inherit)
  Source : ArgOut  DisableCoverage=on  ArgumentName=Source
  Dest : ArgOut  DisableCoverage=on  Port=2  ArgumentName=Dest
  P_s : ArgOut  DisableCoverage=on  Port=3  ArgumentName=P_s
  nqQ : ArgOut  DisableCoverage=on  Port=4  ArgumentName=Q_s
  v : ArgOut  DisableCoverage=on  Port=5  ArgumentName=v
  omega : ArgOut  DisableCoverage=on  Port=6  ArgumentName=omega
  type : ArgOut  DisableCoverage=on  Port=7  ArgumentName=type
  Opt : ArgOut  Port=8  ArgumentName=Opt
  Neighbor_ID : ArgOut  Port=9  ArgumentName=Neighbor_ID
  Neighbor_Opt : ArgOut  Port=10  ArgumentName=Neighbor_Opt
  wires:
  In9/1 -> Neighbor_ID/1  "Neighbor_ID"
  In10/1 -> Neighbor_Opt/1  "Neighbor_Opt"
  Output/1 -> Opt/1  "Opt"
  Input7/1 -> type/1  "type"
  Input5/1 -> omega/1  "omega"
  Input6/1 -> v/1  "v"
  Input4/1 -> nqQ/1  "Q_s"
  Input3/1 -> P_s/1  "P_s"
  Input2/1 -> Dest/1  "Dest"
  Input1/1 -> Source/1  "Source"

== system VFlexP/Grid/Dynamic/Secondary Control/MAS messages/ID1/Simulink Function10 ==
  set_leader : TriggerPort  TriggerType=function-call  IsSimulinkFunction=on  FunctionName=set_leader  FunctionVisibility=scoped  VariantControl=(inherit)
  u : ArgIn  DisableCoverage=on  ArgumentName=u
  Output : Outport
  wires:
  u/1 -> Output/1

== system VFlexP/Grid/Dynamic/Secondary Control/MAS messages/ID1/Simulink Function11 ==
  Input1 : Inport
  get_sending : TriggerPort  TriggerType=function-call  IsSimulinkFunction=on  FunctionName=get_sending  FunctionVisibility=scoped  VariantControl=(inherit)
  value : ArgOut  ArgumentName=value
  wires:
  Input1/1 -> value/1

== system VFlexP/Grid/Dynamic/Secondary Control/MAS messages/ID1/Simulink Function12 ==
  set_sending : TriggerPort  TriggerType=function-call  IsSimulinkFunction=on  FunctionName=set_sending  FunctionVisibility=scoped  VariantControl=(inherit)
  u : ArgIn  DisableCoverage=on  ArgumentName=u
  Output : Outport
  wires:
  u/1 -> Output/1

== system VFlexP/Grid/Dynamic/Secondary Control/MAS messages/ID1/Simulink Function13 ==
  Input1 : Inport
  get_type : TriggerPort  TriggerType=function-call  IsSimulinkFunction=on  FunctionName=get_type  FunctionVisibility=scoped  VariantControl=(inherit)
  value : ArgOut  ArgumentName=type
  wires:
  Input1/1 -> value/1  "type"

== system VFlexP/Grid/Dynamic/Secondary Control/MAS messages/ID1/Simulink Function14 ==
  set_cost_info : TriggerPort  TriggerType=function-call  IsSimulinkFunction=on  FunctionName=set_cost_info  FunctionVisibility=scoped  VariantControl=(inherit)
  cost : ArgIn  ArgumentName=cost
  Output : Outport
  wires:
  cost/1 -> Output/1

== system VFlexP/Grid/Dynamic/Secondary Control/MAS messages/ID1/Simulink Function15 ==
  set_DG_up : TriggerPort  TriggerType=function-call  IsSimulinkFunction=on  FunctionName=set_DG_up  FunctionVisibility=scoped  VariantControl=(inherit)
  u : ArgIn  DisableCoverage=on  ArgumentName=u
  Output : Outport
  wires:
  u/1 -> Output/1

== system VFlexP/Grid/Dynamic/Secondary Control/MAS messages/ID1/Simulink Function16 ==
  Input1 : Inport
  get_DG_up : TriggerPort  TriggerType=function-call  IsSimulinkFunction=on  FunctionName=get_DG_up  FunctionVisibility=scoped  VariantControl=(inherit)
  value : ArgOut  OutDataTypeStr=boolean  ArgumentName=value
  wires:
  Input1/1 -> value/1

== system VFlexP/Grid/Dynamic/Secondary Control/MAS messages/ID1/Simulink Function17 ==
  set_neigh_ID : TriggerPort  TriggerType=function-call  IsSimulinkFunction=on  FunctionName=set_neigh_ID  FunctionVisibility=scoped  VariantControl=(inherit)
  u : ArgIn  DisableCoverage=on  ArgumentName=u
  Output : Outport
  wires:
  u/1 -> Output/1

== system VFlexP/Grid/Dynamic/Secondary Control/MAS messages/ID1/Simulink Function18 ==
  Input1 : Inport
  get_neigh_ID : TriggerPort  TriggerType=function-call  IsSimulinkFunction=on  FunctionName=get_neigh_ID  FunctionVisibility=scoped  VariantControl=(inherit)
  value : ArgOut  ArgumentName=value
  wires:
  Input1/1 -> value/1

== system VFlexP/Grid/Dynamic/Secondary Control/MAS messages/ID1/Simulink Function19 ==
  set_neigh_Opt : TriggerPort  TriggerType=function-call  IsSimulinkFunction=on  FunctionName=set_neigh_Opt  FunctionVisibility=scoped  VariantControl=(inherit)
  u : ArgIn  DisableCoverage=on  ArgumentName=u
  Output : Outport
  wires:
  u/1 -> Output/1

== system VFlexP/Grid/Dynamic/Secondary Control/MAS messages/ID1/Simulink Function2 ==
  unpackage : TriggerPort  TriggerType=function-call  IsSimulinkFunction=on  FunctionName=unpackage  FunctionVisibility=scoped  VariantControl=(inherit)
  IC1 : InitialCondition
  IC2 : InitialCondition
  IC3 : InitialCondition  Value=v_buses_mod(buses_lf(IDnumber))
  IC4 : InitialCondition
  mpP~ : ArgIn  ArgumentName=P_s
  nqQ~ : ArgIn  Port=2  ArgumentName=Q_s
  v : ArgIn  Port=3  ArgumentName=v
  omega : ArgIn  Port=4  ArgumentName=omega
  Output2 : Outport
  Output3 : Outport  Port=2
  Output4 : Outport  Port=3
  Output5 : Outport  Port=4
  wires:
  omega/1 -> IC4/1  "omega"
  v/1 -> IC3/1  "v"
  nqQ~/1 -> IC2/1  "Q_s"
  mpP~/1 -> IC1/1  "P_s"
  IC1/1 -> Output2/1
  IC2/1 -> Output3/1
  IC4/1 -> Output5/1
  IC3/1 -> Output4/1

== system VFlexP/Grid/Dynamic/Secondary Control/MAS messages/ID1/Simulink Function20 ==
  Input1 : Inport
  get_neigh_Opt : TriggerPort  TriggerType=function-call  IsSimulinkFunction=on  FunctionName=get_neigh_Opt  FunctionVisibility=scoped  VariantControl=(inherit)
  value : ArgOut  ArgumentName=value
  wires:
  Input1/1 -> value/1

== system VFlexP/Grid/Dynamic/Secondary Control/MAS messages/ID1/Simulink Function21 ==
  set_sum_neigh_left : TriggerPort  TriggerType=function-call  IsSimulinkFunction=on  FunctionName=set_sum_neigh_left  FunctionVisibility=scoped  VariantControl=(inherit)
  u : ArgIn  DisableCoverage=on  ArgumentName=u
  Output : Outport
  wires:
  u/1 -> Output/1

== system VFlexP/Grid/Dynamic/Secondary Control/MAS messages/ID1/Simulink Function22 ==
  set_Opt : TriggerPort  TriggerType=function-call  IsSimulinkFunction=on  FunctionName=set_Opt  FunctionVisibility=scoped  VariantControl=(inherit)
  u : ArgIn  DisableCoverage=on  ArgumentName=u
  Output : Outport
  wires:
  u/1 -> Output/1

== system VFlexP/Grid/Dynamic/Secondary Control/MAS messages/ID1/Simulink Function23 ==
  Input1 : Inport
  get_sum_neigh_left : TriggerPort  TriggerType=function-call  IsSimulinkFunction=on  FunctionName=get_sum_neigh_left  FunctionVisibility=scoped  VariantControl=(inherit)
  value : ArgOut  ArgumentName=value
  wires:
  Input1/1 -> value/1  "sum_neigh_left"

== system VFlexP/Grid/Dynamic/Secondary Control/MAS messages/ID1/Simulink Function24 ==
  set_decision_turn : TriggerPort  TriggerType=function-call  IsSimulinkFunction=on  FunctionName=set_decision_turn  FunctionVisibility=scoped  VariantControl=(inherit)
  u : ArgIn  DisableCoverage=on  ArgumentName=u
  Output : Outport
  wires:
  u/1 -> Output/1

== system VFlexP/Grid/Dynamic/Secondary Control/MAS messages/ID1/Simulink Function25 ==
  Input1 : Inport
  get_ID : TriggerPort  TriggerType=function-call  IsSimulinkFunction=on  FunctionName=get_ID  FunctionVisibility=scoped  VariantControl=(inherit)
  value : ArgOut  ArgumentName=value
  wires:
  Input1/1 -> value/1

== system VFlexP/Grid/Dynamic/Secondary Control/MAS messages/ID1/Simulink Function26 ==
  set_Neighbor_ID : TriggerPort  TriggerType=function-call  IsSimulinkFunction=on  FunctionName=set_Neighbor_ID  FunctionVisibility=scoped  VariantControl=(inherit)
  u : ArgIn  DisableCoverage=on  ArgumentName=u
  Output : Outport
  wires:
  u/1 -> Output/1

== system VFlexP/Grid/Dynamic/Secondary Control/MAS messages/ID1/Simulink Function27 ==
  set_original_Opt : TriggerPort  TriggerType=function-call  IsSimulinkFunction=on  FunctionName=set_original_Opt  FunctionVisibility=scoped  VariantControl=(inherit)
  u : ArgIn  DisableCoverage=on  ArgumentName=u
  Output : Outport
  wires:
  u/1 -> Output/1

== system VFlexP/Grid/Dynamic/Secondary Control/MAS messages/ID1/Simulink Function28 ==
  set_Neighbor_Opt : TriggerPort  TriggerType=function-call  IsSimulinkFunction=on  FunctionName=set_Neighbor_Opt  FunctionVisibility=scoped  VariantControl=(inherit)
  u : ArgIn  DisableCoverage=on  ArgumentName=u
  Output : Outport
  wires:
  u/1 -> Output/1

== system VFlexP/Grid/Dynamic/Secondary Control/MAS messages/ID1/Simulink Function29 ==
  Input1 : Inport
  get_original_Opt : TriggerPort  TriggerType=function-call  IsSimulinkFunction=on  FunctionName=get_original_Opt  FunctionVisibility=scoped  VariantControl=(inherit)
  value : ArgOut  ArgumentName=value
  wires:
  Input1/1 -> value/1

== system VFlexP/Grid/Dynamic/Secondary Control/MAS messages/ID1/Simulink Function3 ==
  Input1 : Inport
  get_following : TriggerPort  TriggerType=function-call  IsSimulinkFunction=on  FunctionName=get_following  FunctionVisibility=scoped  VariantControl=(inherit)
  value : ArgOut  ArgumentName=value
  wires:
  Input1/1 -> value/1

== system VFlexP/Grid/Dynamic/Secondary Control/MAS messages/ID1/Simulink Function30 ==
  set_original_ID : TriggerPort  TriggerType=function-call  IsSimulinkFunction=on  FunctionName=set_original_ID  FunctionVisibility=scoped  VariantControl=(inherit)
  u : ArgIn  DisableCoverage=on  ArgumentName=u
  Output : Outport
  wires:
  u/1 -> Output/1

== system VFlexP/Grid/Dynamic/Secondary Control/MAS messages/ID1/Simulink Function31 ==
  Input1 : Inport
  get_original_ID : TriggerPort  TriggerType=function-call  IsSimulinkFunction=on  FunctionName=get_original_ID  FunctionVisibility=scoped  VariantControl=(inherit)
  value : ArgOut  ArgumentName=value
  wires:
  Input1/1 -> value/1

== system VFlexP/Grid/Dynamic/Secondary Control/MAS messages/ID1/Simulink Function32 ==
  set_asked : TriggerPort  TriggerType=function-call  IsSimulinkFunction=on  FunctionName=set_asked  FunctionVisibility=scoped  VariantControl=(inherit)
  u : ArgIn  DisableCoverage=on  ArgumentName=u
  Output : Outport
  wires:
  u/1 -> Output/1

== system VFlexP/Grid/Dynamic/Secondary Control/MAS messages/ID1/Simulink Function33 ==
  Input : Inport
  get_cost_P : TriggerPort  TriggerType=function-call  IsSimulinkFunction=on  FunctionName=get_cost_P  FunctionVisibility=scoped  VariantControl=(inherit)
  y : ArgOut  DisableCoverage=on  ArgumentName=y
  wires:
  Input/1 -> y/1

== system VFlexP/Grid/Dynamic/Secondary Control/MAS messages/ID1/Simulink Function34 ==
  Input1 : Inport
  get_asked : TriggerPort  TriggerType=function-call  IsSimulinkFunction=on  FunctionName=get_asked  FunctionVisibility=scoped  VariantControl=(inherit)
  value : ArgOut  ArgumentName=value
  wires:
  Input1/1 -> value/1
